simulink model "Flight_Model_2015a_07_25_2020"  (R2020b)
settings: Solver=ode45  StartTime=0.0  StopTime=100  RelTol=1e-3  EnableMultiTasking=on
model workspace (MAT data in the model file):
  bodyLength = 5
  brakesCd = 1
  brakesOn = 1
  dryCG = 1.9
  dryMass = 23
  finArea = 0.2
  finChordAngle = 0.5236
  finSpan = 0.4
  fullBrakesOn = 0
  gravity = 9.8067
  noseLength = 0.5
  propMass = 7.183
  refArea = 0.0182
  rocketCP = 1
  rocketDiam = 0.197
  targetAlt = 3048
  thrust = [0 2638.366 2528.97 3063.078 2426.009 2548.275 2599.755 2554.71 2644.801 2638.366 2561.145 2606.19 ... (27 elements, 27x1)]
  time = [0 0.045 0.067 0.084 0.124 0.186 0.231 0.298 0.371 0.534 0.979 1.142 ... (27 elements, 27x1)]
  totalImpulse = 10831
  vehicleCd = 0.8
  wetCG = 2.1
  wetMass = 30
undefined symbols (not defined in the file): Earth, WGS84, X, Y, Z
libraries: sm_lib x19, nesl_utility x10, aerolibasang x4, commchan3 x3, simulink x2, aerolibbdyn x2, aerolibwind2 x2, shared6dof x2, shared3dof x1, aerolibtransform2 x1, aerolibfltsims x1, aerolibatmos2 x1
(part 2 of 2)

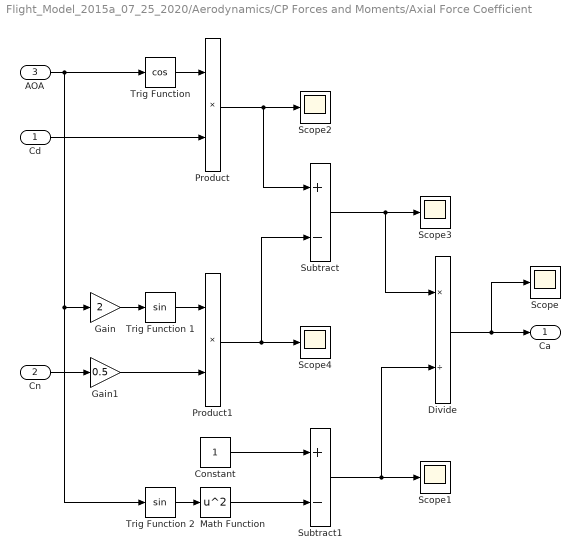
== system Flight_Model_2015a_07_25_2020/Aerodynamics/CP Forces and Moments/Axial Force Coefficient ==
  Cd : Inport
  Cn : Inport  Port=2
  AOA : Inport  Port=3
  Constant : Constant
  Divide : Product  Inputs=*/
  Gain : Gain  Gain=2
  Gain1 : Gain  Gain=0.5
  Math Function : Math  Operator=square  SignedPower=on  SaturateOnIntegerOverflow=on
  Product : Product
  Product1 : Product
  Scope{,1..4} (5 alike) : Scope
  Subtract : Sum  Inputs=+-
  Subtract1 : Sum  Inputs=+-
  Trig Function : Trigonometry  Operator=cos
  Trig Function 1 : Trigonometry
  Trig Function 2 : Trigonometry
  Ca : Outport
  wires:
  AOA/1 -> Trig Function/1, Trig Function 2/1, Gain/1
  Cd/1 -> Product/2
  Trig Function/1 -> Product/1
  Gain/1 -> Trig Function 1/1
  Trig Function 1/1 -> Product1/1
  Gain1/1 -> Product1/2
  Cn/1 -> Gain1/1
  Product1/1 -> Scope4/1, Subtract/2
  Divide/1 -> Scope/1, Ca/1
  Trig Function 2/1 -> Math Function/1
  Math Function/1 -> Subtract1/2
  Constant/1 -> Subtract1/1
  Subtract/1 -> Scope3/1, Divide/1
  Subtract1/1 -> Scope1/1, Divide/2
  Product/1 -> Scope2/1, Subtract/1

== system Flight_Model_2015a_07_25_2020/Aerodynamics/CP Forces and Moments/Axial Force Coefficient1 ==
  Cd : Inport
  AOA : Inport  Port=2
  Product : Product
  Scope : Scope
  Trig Function : Trigonometry  Operator=cos
  Ca : Outport
  wires:
  AOA/1 -> Trig Function/1
  Cd/1 -> Product/2
  Trig Function/1 -> Product/1
  Product/1 -> Ca/1, Scope/1

== system Flight_Model_2015a_07_25_2020/Aerodynamics/CP Forces and Moments/Axial Forces ==
  Ca : Inport
  Aref : Inport  Port=2
  "q " : Inport  Port=3
  Product : Product  Inputs=3
  Scope : Scope
  Axial Force : Outport
  wires:
  Ca/1 -> Product/1
  Aref/1 -> Product/2
  Product/1 -> Axial Force/1, Scope/1
  "q "/1 -> Product/3

== system Flight_Model_2015a_07_25_2020/Aerodynamics/CP Forces and Moments/Drag Force Coefficient ==
  In1 : Inport
  Cd : Outport
  wires:
  In1/1 -> Cd/1

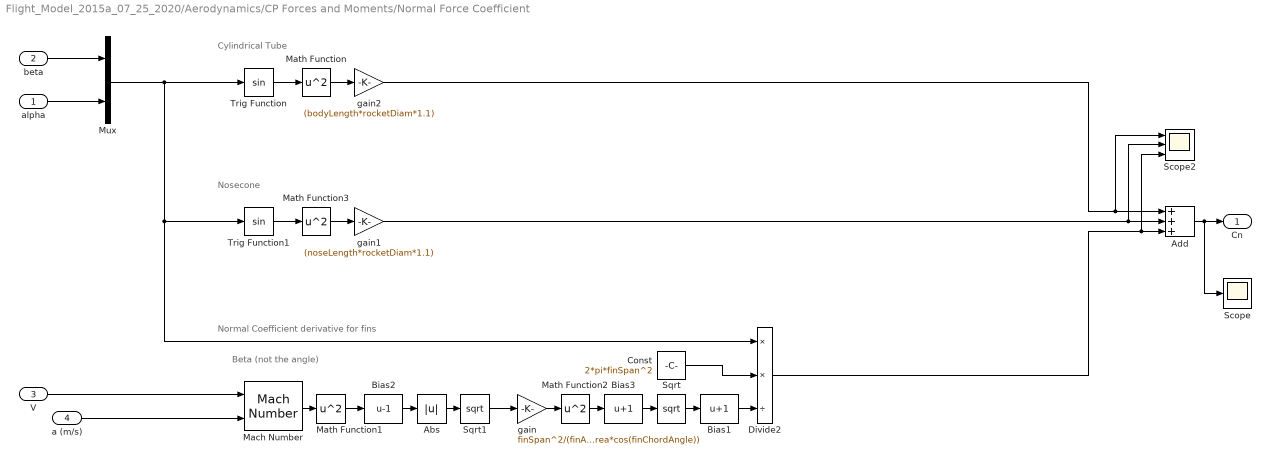
== system Flight_Model_2015a_07_25_2020/Aerodynamics/CP Forces and Moments/Normal Force Coefficient ==
  note: Cylindrical Tube
  note: Normal Coefficient derivative for fins
  note: Beta (not the angle)
  note: Nosecone
  alpha : Inport
  beta : Inport  Port=2
  V : Inport  Port=3
  a (m/s) : Inport  Port=4
  Abs : Abs
  Add : Sum  Inputs=+++
  Bias1 : Bias  Bias=1
  Bias2 : Bias  Bias=-1
  Bias3 : Bias  Bias=1
  Const : Constant  Value=2*pi*finSpan^2
  Divide2 : Product  Inputs=**/
  Mach Number : aerolibasang/Mach Number
      settings: SourceProductBaseCode=AE
  Math Function{,1..3} (4 alike) : Math  Operator=square  SignedPower=on  SaturateOnIntegerOverflow=on
  Mux : Mux  Inputs=2
  Scope : Scope
  Scope2 : Scope  NumInputPorts=3
  Sqrt : Sqrt  SaturateOnIntegerOverflow=on
  Sqrt1 : Sqrt  SaturateOnIntegerOverflow=on
  Trig Function : Trigonometry
  Trig Function1 : Trigonometry
  gain : Gain  Gain=finSpan^2/(finArea*cos(finChordAngle))
  gain1 : Gain  Gain=(noseLength*rocketDiam*1.1)
  gain2 : Gain  Gain=(bodyLength*rocketDiam*1.1)
  Cn : Outport
  wires:
  Trig Function/1 -> Math Function/1
  Sqrt1/1 -> gain/1
  Math Function2/1 -> Bias3/1
  Sqrt/1 -> Bias1/1
  Bias3/1 -> Sqrt/1
  gain/1 -> Math Function2/1
  a (m/s)/1 -> Mach Number/2
  Bias1/1 -> Divide2/3
  Math Function/1 -> gain2/1
  Trig Function1/1 -> Math Function3/1
  Math Function3/1 -> gain1/1
  Add/1 -> Scope/1, Cn/1
  V/1 -> Mach Number/1
  Mach Number/1 -> Math Function1/1
  Math Function1/1 -> Bias2/1
  Bias2/1 -> Abs/1
  Abs/1 -> Sqrt1/1
  Mux/1 -> Divide2/1, Trig Function1/1, Trig Function/1
  Const/1 -> Divide2/2
  gain1/1 -> Scope2/2, Add/2
  gain2/1 -> Add/1, Scope2/1
  Divide2/1 -> Add/3, Scope2/3
  alpha/1 -> Mux/2
  beta/1 -> Mux/1

== system Flight_Model_2015a_07_25_2020/Aerodynamics/CP Forces and Moments/Normal Forces ==
  Cn : Inport
  Aref : Inport  Port=2
  "q " : Inport  Port=3
  Product : Product  Inputs=3
  Scope : Scope
  Normal Force : Outport
  wires:
  Cn/1 -> Product/1
  Aref/1 -> Product/2
  Product/1 -> Normal Force/1, Scope/1
  "q "/1 -> Product/3

== system Flight_Model_2015a_07_25_2020/Avionics/Pressure Sensor/Pressure to Altitude ==
  note: \/ \/ to power of 1/5.257
  note: presser & temp to altitude
  Atmostpheric Pressure : Inport
  "Temp (C) " : Inport  Port=2
  Add : Sum
  Constant : Constant  Value=273.15
  Constant1 : Constant  Value=.0065
  Constant2 : Constant
  Divide : Product  Inputs=*/
  Divide1 : Product  Inputs=*/
  Fcn : Fcn  Expr=u^0.19022256039
  Product : Product
  Subtract : Sum  Inputs=+-
  sealevel pressure : Constant  Value=1013.25
  Altitude : Outport
  wires:
  Constant/1 -> Add/2
  "Temp (C) "/1 -> Add/1
  Constant1/1 -> Divide/2
  Constant2/1 -> Subtract/2
  Add/1 -> Product/2
  Atmostpheric Pressure/1 -> Divide1/2
  sealevel pressure/1 -> Divide1/1
  Divide/1 -> Altitude/1
  Subtract/1 -> Product/1
  Product/1 -> Divide/1
  Fcn/1 -> Subtract/1
  Divide1/1 -> Fcn/1
